simulink model "util_thruster_hrn"  (R2014b)
settings: Solver=FixedStepDiscrete  StartTime=0.0  StopTime=1  FixedStep=1  RelTol=1e-3
libraries: util_thruster_lib x7
settings Model: RequirementInfo={'other' 'util_thruster_req.html' '' 'true' 'Requirements for Thruster models' ' util_thruster_0001' } %GIDa_9a73fb04_1174_49ad_89b1_633e90eb97d3  ExtModeAutoUpdateStatusClock=off  Creator=hcannon  LastModifiedBy=mstewart
settings DataIOCC: SignalLoggingSaveFormat=ModelDataLogs
settings OptimizationCC: ExpressionDepthLimit=2147483647  InitFltsAndDblsToZero=on
settings DebuggingCC: UnderspecifiedInitializationDetection=Classic  MergeDetectMultiDrivingBlocksExec=none  FcnCallInpInsideContextMsg=UseLocalSettings  StateNameClashWarn=warning  StrictBusMsg=Warning
settings GRTTargetCC: CombineOutputUpdateFcns=off  GRTInterface=on

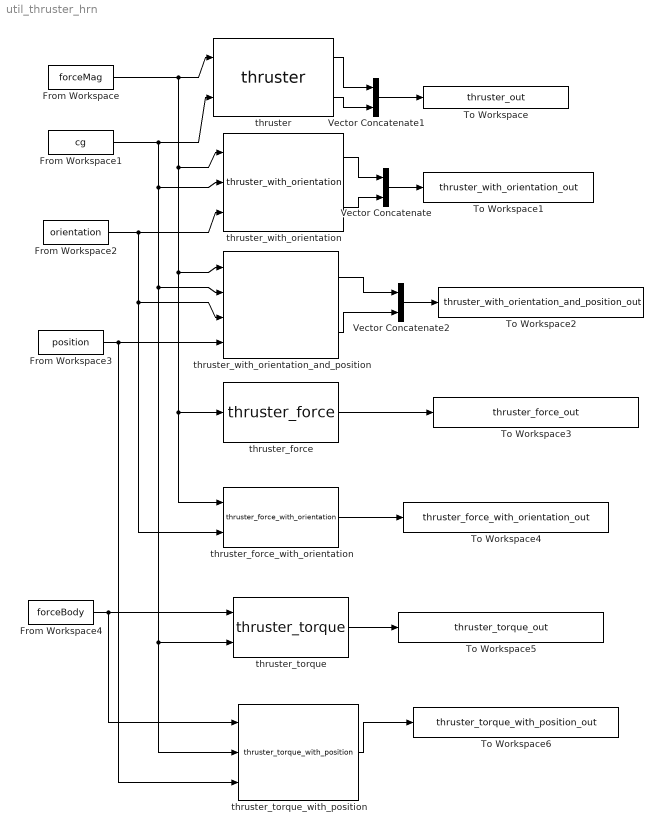
== system util_thruster_hrn ==
  From Workspace : FromWorkspace  VariableName=forceMag  SampleTime=0
  From Workspace1 : FromWorkspace  VariableName=cg  SampleTime=0
  From Workspace2 : FromWorkspace  VariableName=orientation  SampleTime=0
  From Workspace3 : FromWorkspace  VariableName=position  SampleTime=0
  From Workspace4 : FromWorkspace  VariableName=forceBody  SampleTime=0
  To Workspace : ToWorkspace  VariableName=thruster_out  SampleTime=-1
  To Workspace1 : ToWorkspace  VariableName=thruster_with_orientation_out  SampleTime=-1
  To Workspace2 : ToWorkspace  VariableName=thruster_with_orientation_and_position_out  SampleTime=-1
  To Workspace3 : ToWorkspace  VariableName=thruster_force_out  SampleTime=-1
  To Workspace4 : ToWorkspace  VariableName=thruster_force_with_orientation_out  SampleTime=-1
  To Workspace5 : ToWorkspace  VariableName=thruster_torque_out  SampleTime=-1
  To Workspace6 : ToWorkspace  VariableName=thruster_torque_with_position_out  SampleTime=-1
  Vector Concatenate : Concatenate
  Vector Concatenate1 : Concatenate
  Vector Concatenate2 : Concatenate
  thruster : util_thruster_lib/thruster  Thruster_Position=positionP  Thruster_Orientation=orientationP
  thruster_force : util_thruster_lib/thruster_force  Thruster_Orientation=orientationP
  thruster_force_with_orientation : util_thruster_lib/thruster_force_with_orientation
  thruster_torque : util_thruster_lib/thruster_torque  Thruster_Position=positionP
  thruster_torque_with_position : util_thruster_lib/thruster_torque_with_position
  thruster_with_orientation : util_thruster_lib/thruster_with_orientation  Thruster_Position=positionP
  thruster_with_orientation_and_position : util_thruster_lib/thruster_with_orientation_and_position
  wires:
  From Workspace/1 -> thruster/1, thruster_with_orientation/1, thruster_with_orientation_and_position/1, thruster_force/1, thruster_force_with_orientation/1
  From Workspace1/1 -> thruster/2, thruster_with_orientation/2, thruster_with_orientation_and_position/2, thruster_torque/2, thruster_torque_with_position/2
  From Workspace2/1 -> thruster_with_orientation/3, thruster_with_orientation_and_position/3, thruster_force_with_orientation/2
  From Workspace3/1 -> thruster_with_orientation_and_position/4, thruster_torque_with_position/3
  thruster/1 -> Vector Concatenate1/1
  thruster/2 -> Vector Concatenate1/2
  Vector Concatenate1/1 -> To Workspace/1
  thruster_with_orientation/1 -> Vector Concatenate/1
  thruster_with_orientation/2 -> Vector Concatenate/2
  Vector Concatenate/1 -> To Workspace1/1
  thruster_with_orientation_and_position/1 -> Vector Concatenate2/1
  thruster_with_orientation_and_position/2 -> Vector Concatenate2/2
  Vector Concatenate2/1 -> To Workspace2/1
  thruster_force/1 -> To Workspace3/1
  thruster_force_with_orientation/1 -> To Workspace4/1
  thruster_torque/1 -> To Workspace5/1
  thruster_torque_with_position/1 -> To Workspace6/1
  From Workspace4/1 -> thruster_torque/1, thruster_torque_with_position/1
